simulink model "gm_untitled"  (R2020a)
settings: Solver=FixedStepDiscrete  StartTime=0.0  StopTime=10  RelTol=1e-3
settings Model: Creator=572170017@qq.com  LastModifiedBy=572170017@qq.com
settings DataIOCC: LimitDataPoints=on  SaveOutput=off  SignalLogging=off  SaveTime=off
settings OptimizationCC: BlockReduction=off  ConditionallyExecuteInputs=off  DefaultParameterBehavior=Inlined  ExpressionDepthLimit=2147483647  LifeSpan=inf
settings DebuggingCC: AlgebraicLoopMsg=error  UnderspecifiedInitializationDetection=Classic  MergeDetectMultiDrivingBlocksExec=none  InheritedTsInSrcMsg=none  SingleTaskRateTransMsg=error  ParameterPrecisionLossMsg=none  AllowSymbolicDim=off  StateNameClashWarn=warning  StrictBusMsg=ErrorOnBusTreatedAsVector  SFUnexpectedBacktrackingDiag=warning  SFNoUnconditionalDefaultTransitionDiag=warning  SFExecutionAtInitializationDiag=none  ArithmeticOperatorsInVariantConditions=warning
settings HardwareCC: ProdBitPerPointer=32  ProdBitPerSizeT=32  ProdBitPerPtrDiffT=32  ProdLargestAtomicFloat=None  ProdIntDivRoundTo=Undefined  ProdEndianess=Unspecified  ProdWordSize=32  ProdHWDeviceType=ASIC/FPGA->ASIC/FPGA  ProdEqTarget=off
settings SFSimCC: SimUseLocalCustomCode=off  CustomCodeUndefinedFunction=UseInterfaceOnly
settings RTWCC: RTWUseLocalCustomCode=off
settings CodeAppCC: StateflowObjectComments=on
settings GRTTargetCC: TargetLangStandard=C89/C90 (ANSI)
settings ConfigComp: CovScope=ReferencedModels  CovMetricSettings=dw  CovHtmlReporting=on  CovSaveCumulativeToWorkspaceVar=on  CovSaveSingleToWorkspaceVar=on  CovExternalEMLEnable=off  CovSFcnEnable=off

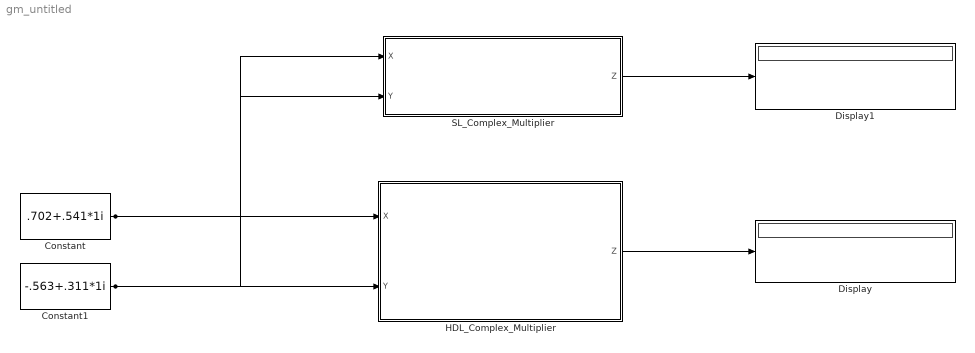
== system gm_untitled ==
  Constant : Constant  Value=.702+.541*1i  VectorParams1D=off  OutDataTypeStr=fixdt(1,18,17)  SampleTime=1
  Constant1 : Constant  Value=-.563+.311*1i  VectorParams1D=off  OutDataTypeStr=fixdt(1,18,17)  SampleTime=1
  Display : Display
  Display1 : Display
  HDL_Complex_Multiplier : Subsystem
  SL_Complex_Multiplier : Subsystem
  wires:
  SL_Complex_Multiplier/1(Z) -> Display1/1
  Constant1/1 -> HDL_Complex_Multiplier/2(Y), SL_Complex_Multiplier/2(Y)
  Constant/1 -> HDL_Complex_Multiplier/1(X), SL_Complex_Multiplier/1(X)
  HDL_Complex_Multiplier/1(Z) -> Display/1

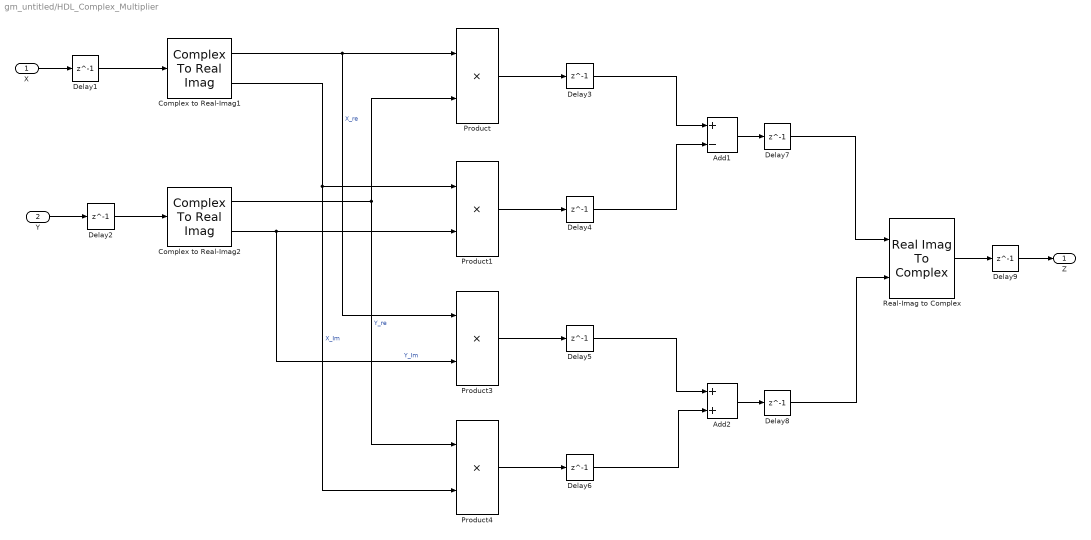
== system gm_untitled/HDL_Complex_Multiplier ==
  X : Inport
  Y : Inport  Port=2
  Add1 : Sum  Inputs=+-
  Add2 : Sum
  Complex to Real-Imag1 : ComplexToRealImag
  Complex to Real-Imag2 : ComplexToRealImag
  Delay{1..9} (9 alike) : Delay  DelayLength=1
  Product{,1,3..4} (4 alike) : Product
  Real-Imag to Complex : RealImagToComplex
  Z : Outport
  wires:
  Delay8/1 -> Real-Imag to Complex/2
  Delay7/1 -> Real-Imag to Complex/1
  Delay5/1 -> Add2/1
  Add2/1 -> Delay8/1
  Delay2/1 -> Complex to Real-Imag2/1
  Delay1/1 -> Complex to Real-Imag1/1
  Delay9/1 -> Z/1
  X/1 -> Delay1/1
  Y/1 -> Delay2/1
  Add1/1 -> Delay7/1
  Delay6/1 -> Add2/2
  Delay4/1 -> Add1/2
  Delay3/1 -> Add1/1
  Complex to Real-Imag1/2 -> Product1/1, Product4/2  "X_Im"
  Complex to Real-Imag2/1 -> Product/2, Product4/1  "Y_re"
  Complex to Real-Imag2/2 -> Product1/2, Product3/2  "Y_Im"
  Complex to Real-Imag1/1 -> Product/1, Product3/1  "X_re"
  Real-Imag to Complex/1 -> Delay9/1
  Product4/1 -> Delay6/1
  Product3/1 -> Delay5/1
  Product1/1 -> Delay4/1
  Product/1 -> Delay3/1

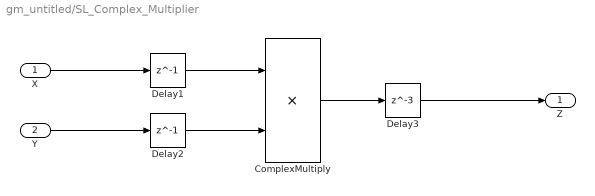
== system gm_untitled/SL_Complex_Multiplier ==
  X : Inport
  Y : Inport  Port=2
  ComplexMultiply : Product  OutDataTypeStr=fixdt(1,37,34)
  Delay1 : Delay  DelayLength=1
  Delay2 : Delay  DelayLength=1
  Delay3 : Delay  DelayLength=3
  Z : Outport
  wires:
  Delay2/1 -> ComplexMultiply/2
  Delay1/1 -> ComplexMultiply/1
  Delay3/1 -> Z/1
  X/1 -> Delay1/1
  Y/1 -> Delay2/1
  ComplexMultiply/1 -> Delay3/1
